simulink model "rov_kinematics_level1"  (R2024b)
settings: Solver=VariableStepAuto  StartTime=0.0  StopTime=90  RelTol=1e-3
settings Model: Creator=eirikvarnes  LastModifiedBy=eirikvarnes
settings DataIOCC: SaveFormat=Array  SaveTime=off  ReturnWorkspaceOutputs=off  OutputSaveName=eta

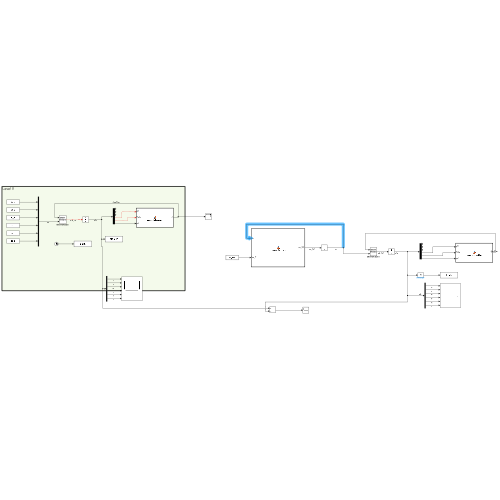
[thumbnail: Simulink's stored preview of the top-level diagram]
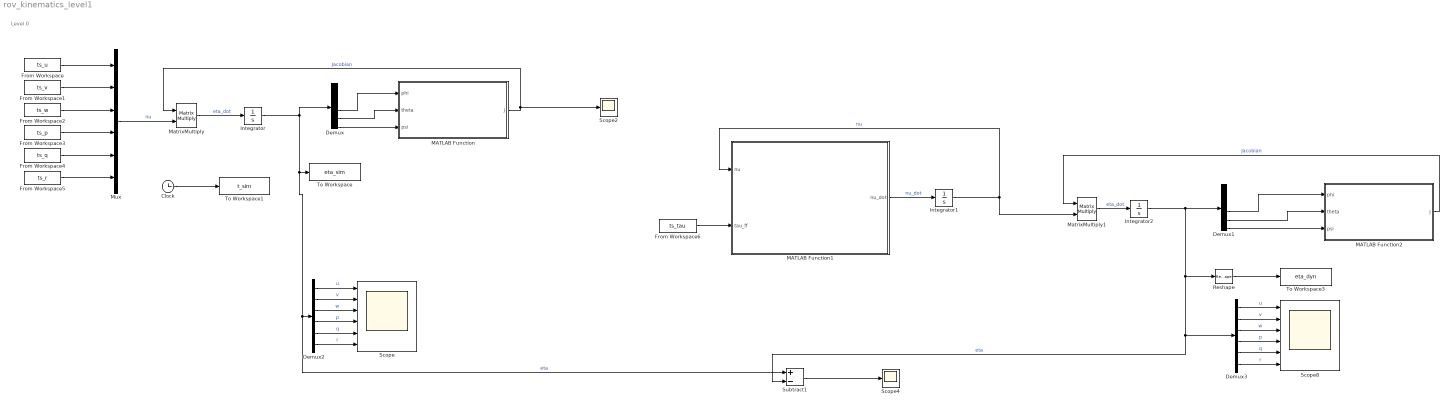
== system rov_kinematics_level1 ==
  note: Level 0
  Clock : Clock
  Demux{,1..3} (4 alike) : Demux  Outputs=6
  From Workspace : FromWorkspace  VariableName=ts_u
  From Workspace1 : FromWorkspace  VariableName=ts_v
  From Workspace2 : FromWorkspace  VariableName=ts_w
  From Workspace3 : FromWorkspace  VariableName=ts_p
  From Workspace4 : FromWorkspace  VariableName=ts_q
  From Workspace5 : FromWorkspace  VariableName=ts_r
  From Workspace6 : FromWorkspace  VariableName=ts_tau  SampleTime=-1
  Integrator : Integrator
  Integrator1 : Integrator
  Integrator2 : Integrator
  MATLAB Function : MATLAB Function  TreatAsAtomicUnit=on
  MATLAB Function1 : MATLAB Function  TreatAsAtomicUnit=on
  MATLAB Function2 : MATLAB Function  TreatAsAtomicUnit=on
  MatrixMultiply : Product  Multiplication=Matrix(*)
  MatrixMultiply1 : Product  Multiplication=Matrix(*)
  Mux : Mux  Inputs=6
  Reshape : Reshape  OutputDimensionality=Customize  OutputDimensions=[1 6]
  Scope : Scope  NumInputPorts=6
  Scope2 : Scope
  Scope4 : Scope
  Scope8 : Scope  NumInputPorts=6
  Subtract1 : Sum  Inputs=+-
  To Workspace : ToWorkspace  VariableName=eta_sim  SampleTime=-1
  To Workspace1 : ToWorkspace  VariableName=t_sim  SampleTime=-1
  To Workspace3 : ToWorkspace  VariableName=eta_dyn  SampleTime=-1
  wires:
  MATLAB Function/1(J) -> Scope2/1, MatrixMultiply/1  "Jacobian"
  Demux/4 -> MATLAB Function/1(phi)
  Demux/5 -> MATLAB Function/2(theta)
  Demux/6 -> MATLAB Function/3(psi)
  Integrator/1 -> Subtract1/1, Demux2/1, To Workspace/1, Demux/1  "eta"
  MatrixMultiply/1 -> Integrator/1  "eta_dot"
  From Workspace/1 -> Mux/1
  From Workspace1/1 -> Mux/2
  From Workspace2/1 -> Mux/3
  From Workspace3/1 -> Mux/4
  From Workspace4/1 -> Mux/5
  From Workspace5/1 -> Mux/6
  Mux/1 -> MatrixMultiply/2  "nu"
  Clock/1 -> To Workspace1/1
  Demux2/1 -> Scope/1  "u"
  Demux2/2 -> Scope/2  "v"
  Demux2/3 -> Scope/3  "w"
  Demux2/4 -> Scope/4  "p"
  Demux2/5 -> Scope/5  "q"
  Demux2/6 -> Scope/6  "r"
  MATLAB Function1/1(nu_dot) -> Integrator1/1  "nu_dot"
  Integrator1/1 -> MatrixMultiply1/2, MATLAB Function1/1(nu)  "nu"
  MATLAB Function2/1(J) -> MatrixMultiply1/1  "Jacobian"
  Demux1/6 -> MATLAB Function2/3(psi)
  Demux1/4 -> MATLAB Function2/1(phi)
  MatrixMultiply1/1 -> Integrator2/1  "eta_dot"
  Demux1/5 -> MATLAB Function2/2(theta)
  Demux3/2 -> Scope8/2  "v"
  Demux3/3 -> Scope8/3  "w"
  Demux3/5 -> Scope8/5  "q"
  Demux3/1 -> Scope8/1  "u"
  Integrator2/1 -> Reshape/1, Subtract1/2, Demux3/1, Demux1/1  "eta"
  Demux3/4 -> Scope8/4  "p"
  Demux3/6 -> Scope8/6  "r"
  Subtract1/1 -> Scope4/1
  From Workspace6/1 -> MATLAB Function1/2(tau_ff)
  Reshape/1 -> To Workspace3/1

== matlab function rov_kinematics_level1/MATLAB Function1 ==
  data: nu input size=[6 1]; tau_ff input; nu_dot output size=[6 1]
function nu_dot = computeDynamics(nu, tau_ff)
% computeDynamics  1st‐order dynamics with added‐mass & damping only
%   nu_dot = M_R^{-1} * (tau_ff - D*nu)
%
%   Inputs nu and tau_ff must both be 6-by-1 vectors.

  %#codegen
  % Verify inputs are 6-by-1
  assert(all(size(nu)==[6,1]),  'computeDynamics:InvalidInput', 'nu must be 6-by-1');
  assert(all(size(tau_ff)==[6,1]), 'computeDynamics:InvalidInput', 'tau_ff must be 6-by-1');

  % Pull in parameters
  params = rovParameters();

  % Total mass + added‐mass
  M_rb = [params.mass*eye(3), zeros(3);
          zeros(3),           params.I];
  M_A  = -diag([params.Ma_lin; params.Ma_rot]);
  M_R  = M_rb + M_A;

  % Damping
  D_lin  = diag(params.D_lin);
  D_quad = diag(params.D_quad .* abs(nu));
  D      = D_lin + D_quad;

  % Dynamics
  nu_dot = M_R \ (tau_ff - D*nu);
end

== matlab function rov_kinematics_level1/MATLAB Function ==
  data: phi input; J output; theta input; psi input
function J = computeJacobian(phi, theta, psi)
% computeJacobian  ZYX‐Euler Jacobian with singularity clamp
%   Inputs:
%     phi, theta, psi  – Euler angles (roll, pitch, yaw), in radians
%   Output:
%     J  – 6×6 Jacobian mapping [u;v;w;p;q;r] to [xdot;ydot;zdot;phidot;thetadot;psidot]

  %#codegen
  % 1) Rotation matrix R = Rz(psi)*Ry(theta)*Rx(phi)
  cphi = cos(phi);   sphi = sin(phi);
  ctheta = cos(theta); stheta = sin(theta);
  cpsi = cos(psi);   spsi = sin(psi);

  Rz = [ cpsi, -spsi, 0;
         spsi,  cpsi, 0;
           0 ,    0 , 1 ];
  Ry = [ ctheta, 0, stheta;
            0  , 1,   0  ;
        -stheta,0, ctheta ];
  Rx = [ 1,   0  ,   0   ;
         0, cphi, -sphi ;
         0, sphi,  cphi ];
  R = Rz * Ry * Rx;

  % 2) Clamp cos(theta) away from zero to avoid singularity
  epsilon = 5e-3;                          % adjust if needed
  safe_ct = max(abs(ctheta), epsilon) * sign(ctheta);

  % 3) Build T matrix for Euler rates
  %    [phidot; thetadot; psidot] = T * [p; q; r]
  T = [ 1,      sphi*(stheta/safe_ct),   cphi*(stheta/safe_ct);
        0,            cphi,                -sphi;
        0,     sphi/safe_ct,             cphi/safe_ct ];

  % 4) Assemble full Jacobian
  J = [ R,          zeros(3,3);
        zeros(3,3), T       ];
end

== matlab function rov_kinematics_level1/MATLAB Function2 ==
  data: phi input; J output; theta input; psi input
function J = computeJacobian(phi, theta, psi)
% computeJacobian  ZYX‐Euler Jacobian with singularity clamp
%   Inputs:
%     phi, theta, psi  – Euler angles (roll, pitch, yaw), in radians
%   Output:
%     J  – 6×6 Jacobian mapping [u;v;w;p;q;r] to [xdot;ydot;zdot;phidot;thetadot;psidot]

  %#codegen
  % 1) Rotation matrix R = Rz(psi)*Ry(theta)*Rx(phi)
  cphi = cos(phi);   sphi = sin(phi);
  ctheta = cos(theta); stheta = sin(theta);
  cpsi = cos(psi);   spsi = sin(psi);

  Rz = [ cpsi, -spsi, 0;
         spsi,  cpsi, 0;
           0 ,    0 , 1 ];
  Ry = [ ctheta, 0, stheta;
            0  , 1,   0  ;
        -stheta,0, ctheta ];
  Rx = [ 1,   0  ,   0   ;
         0, cphi, -sphi ;
         0, sphi,  cphi ];
  R = Rz * Ry * Rx;

  % 2) Clamp cos(theta) away from zero to avoid singularity
  epsilon = 5e-3;                          % adjust if needed
  safe_ct = max(abs(ctheta), epsilon) * sign(ctheta);

  % 3) Build T matrix for Euler rates
  %    [phidot; thetadot; psidot] = T * [p; q; r]
  T = [ 1,      sphi*(stheta/safe_ct),   cphi*(stheta/safe_ct);
        0,            cphi,                -sphi;
        0,     sphi/safe_ct,             cphi/safe_ct ];

  % 4) Assemble full Jacobian
  J = [ R,          zeros(3,3);
        zeros(3,3), T       ];
end
